simulink model "controller_estimator_test_static"  (R2016b)
settings: Solver=VariableStepAuto  StartTime=0.0  StopTime=200  RelTol=1e-3
values from neighbouring files (symbols this model uses):
  quat_cmd = quat_cmd/norm(quat_cmd)    [controller_estimator_test_init.m]
undefined symbols (not defined in the file or in its folder): Estimation_EKF, extended_kalman_filter_lib, fsw_params
libraries: dynamics_lib x2, pd_control_lib x1, aerolibutil x1, sensors_lib x1, sensor_processing x1
settings Model: Creator=sexymathemagician  LastModifiedBy=sexymathemagician

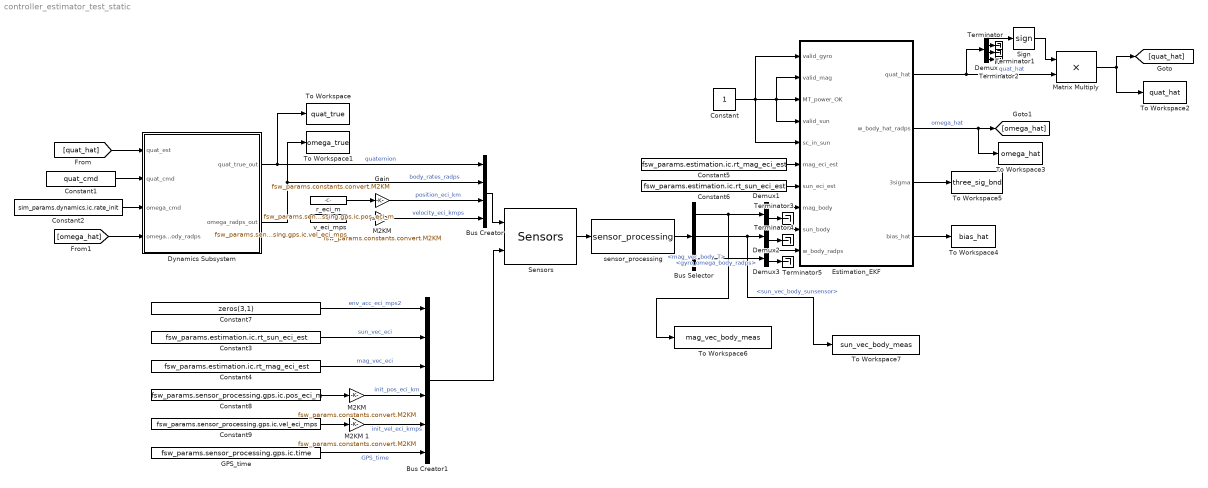
== system controller_estimator_test_static ==
  Bus Creator : BusCreator  Inputs=4
  Bus Creator1 : BusCreator  Inputs=6
  Bus Selector : BusSelector  OutputSignals=mag_vec_body_T,sun_vec_body_sunsensor,gyro_omega_body_radps
  Constant : Constant
  Constant1 : Constant  Value=quat_cmd
  Constant2 : Constant  Value=sim_params.dynamics.ic.rate_init
  Constant3 : Constant  Value=fsw_params.estimation.ic.rt_sun_eci_est
  Constant4 : Constant  Value=fsw_params.estimation.ic.rt_mag_eci_est
  Constant5 : Constant  Value=fsw_params.estimation.ic.rt_mag_eci_est
  Constant6 : Constant  Value=fsw_params.estimation.ic.rt_sun_eci_est
  Constant7 : Constant  Value=zeros(3,1)
  Constant8 : Constant  Value=fsw_params.sensor_processing.gps.ic.pos_eci_m
  Constant9 : Constant  Value=fsw_params.sensor_processing.gps.ic.vel_eci_mps
  Demux : Demux
  Demux1 : Demux  Outputs=[3 1]
  Demux2 : Demux  Outputs=[3 1]
  Demux3 : Demux  Outputs=[3 1]
  Dynamics Subsystem : Subsystem
  "Estimation_EKF " : Subsystem  AncestorBlock=extended_kalman_filter_lib/Estimation_EKF
  GPS_time : Constant  Value=fsw_params.sensor_processing.gps.ic.time
  Gain : Gain  Gain=fsw_params.constants.convert.M2KM
  M2KM : Gain  Gain=fsw_params.constants.convert.M2KM
  "M2KM " : Gain  Gain=fsw_params.constants.convert.M2KM
  M2KM 1 : Gain  Gain=fsw_params.constants.convert.M2KM
  Matrix Multiply : Product
  Sensors : sensors_lib/Sensors
      link override Bus Selector2: OutputSignals=sun_vec_eci,mag_vec_eci
  Sign : Signum
  Terminator{,1..5} (6 alike) : Terminator
  To Workspace : ToWorkspace  VariableName=quat_true  SaveFormat=Timeseries  SampleTime=-1
  To Workspace1 : ToWorkspace  VariableName=omega_true  SaveFormat=Timeseries  SampleTime=-1
  To Workspace2 : ToWorkspace  VariableName=quat_hat  SaveFormat=Timeseries  SampleTime=-1
  To Workspace3 : ToWorkspace  VariableName=omega_hat  SaveFormat=Timeseries  SampleTime=-1
  To Workspace4 : ToWorkspace  VariableName=bias_hat  SaveFormat=Timeseries  SampleTime=-1
  To Workspace5 : ToWorkspace  VariableName=three_sig_bnd  SaveFormat=Timeseries  SampleTime=-1
  To Workspace6 : ToWorkspace  VariableName=mag_vec_body_meas  SaveFormat=Timeseries  SampleTime=-1
  To Workspace7 : ToWorkspace  VariableName=sun_vec_body_meas  SaveFormat=Timeseries  SampleTime=-1
  r_eci_m : Constant  Value=fsw_params.sensor_processing.gps.ic.pos_eci_m
  sensor_processing : sensor_processing/sensor_processing
  v_eci_mps : Constant  Value=fsw_params.sensor_processing.gps.ic.vel_eci_mps
  wires:
  Constant/1 -> "Estimation_EKF "/5(sc_in_sun), "Estimation_EKF "/1(valid_gyro), "Estimation_EKF "/4("valid_sun "), "Estimation_EKF "/2(valid_mag), "Estimation_EKF "/3(MT_power_OK)
  "Estimation_EKF "/3(3sigma) -> To Workspace5/1
  "Estimation_EKF "/4(bias_hat) -> To Workspace4/1
  Dynamics Subsystem/1(quat_true_out) -> Bus Creator/1, To Workspace/1  "quaternion"
  Dynamics Subsystem/2(omega_radps_out) -> Bus Creator/2, To Workspace1/1  "body_rates_radps"
  [quat_hat] -> Dynamics Subsystem/1(quat_est)
  "Estimation_EKF "/2(w_body_hat_radps) -> To Workspace3/1, [omega_hat]  "omega_hat"
  [omega_hat] -> Dynamics Subsystem/4(omega_body_radps)
  Constant1/1 -> Dynamics Subsystem/2(quat_cmd)
  Constant2/1 -> Dynamics Subsystem/3("omega_cmd ")
  "Estimation_EKF "/1(quat_hat) -> Demux/1, Matrix Multiply/2  "quat_hat"
  Demux/2 -> Terminator/1
  Demux/3 -> Terminator1/1
  Demux/4 -> Terminator2/1
  Demux/1 -> Sign/1
  Sign/1 -> Matrix Multiply/1
  Sensors/1 -> sensor_processing/1
  sensor_processing/1 -> Bus Selector/1
  Bus Creator/1 -> Sensors/1
  Bus Selector/1 -> To Workspace6/1, Demux1/1  "<mag_vec_body_T>"
  Bus Selector/2 -> To Workspace7/1, Demux2/1  "<sun_vec_body_sunsensor>"
  Bus Selector/3 -> Demux3/1  "<gyro_omega_body_radps>"
  r_eci_m/1 -> Gain/1
  Constant4/1 -> Bus Creator1/3  "mag_vec_eci"
  Constant3/1 -> Bus Creator1/2  "sun_vec_eci"
  GPS_time/1 -> Bus Creator1/6  "GPS_time"
  Bus Creator1/1 -> Sensors/2
  Constant6/1 -> "Estimation_EKF "/7(sun_eci_est)
  Constant5/1 -> "Estimation_EKF "/6(mag_eci_est)
  Constant7/1 -> Bus Creator1/1  "env_acc_eci_mps2"
  Constant8/1 -> "M2KM "/1
  Constant9/1 -> M2KM 1/1
  Gain/1 -> Bus Creator/3  "position_eci_km"
  v_eci_mps/1 -> M2KM/1
  M2KM/1 -> Bus Creator/4  "velocity_eci_kmps"
  "M2KM "/1 -> Bus Creator1/4  "init_pos_eci_km"
  M2KM 1/1 -> Bus Creator1/5  "init_vel_eci_kmps"
  Demux1/1 -> "Estimation_EKF "/8(mag_body)
  Demux2/1 -> "Estimation_EKF "/9(sun_body)
  Demux3/1 -> "Estimation_EKF "/10(w_body_radps)
  Demux1/2 -> Terminator3/1
  Demux2/2 -> Terminator4/1
  Demux3/2 -> Terminator5/1
  Matrix Multiply/1 -> To Workspace2/1, [quat_hat]

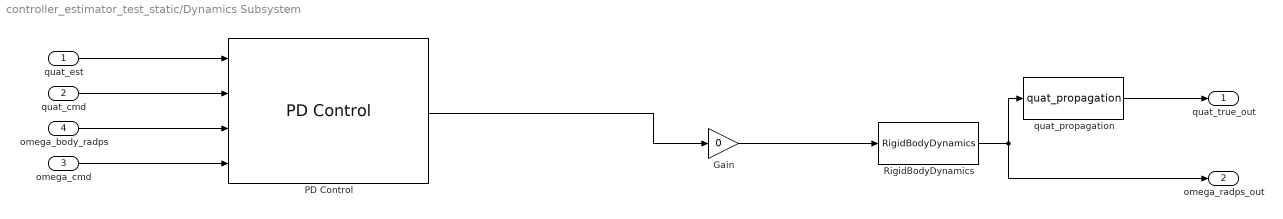
== system controller_estimator_test_static/Dynamics Subsystem ==
  quat_est : Inport
  quat_cmd : Inport  Port=2
  "omega_cmd " : Inport  Port=3
  omega_body_radps : Inport  Port=4
  Gain : Gain  Gain=0
  PD Control : pd_control_lib/PD Control
  RigidBodyDynamics : dynamics_lib/Dynamics/RigidBodyDynamics
  quat_propagation : dynamics_lib/Dynamics/quat_propagation
  quat_true_out : Outport
  omega_radps_out : Outport  Port=2
  wires:
  "omega_cmd "/1 -> PD Control/4
  quat_est/1 -> PD Control/1
  quat_cmd/1 -> PD Control/2
  omega_body_radps/1 -> PD Control/3
  RigidBodyDynamics/1 -> omega_radps_out/1, quat_propagation/1
  quat_propagation/1 -> quat_true_out/1
  PD Control/1 -> Gain/1
  Gain/1 -> RigidBodyDynamics/1

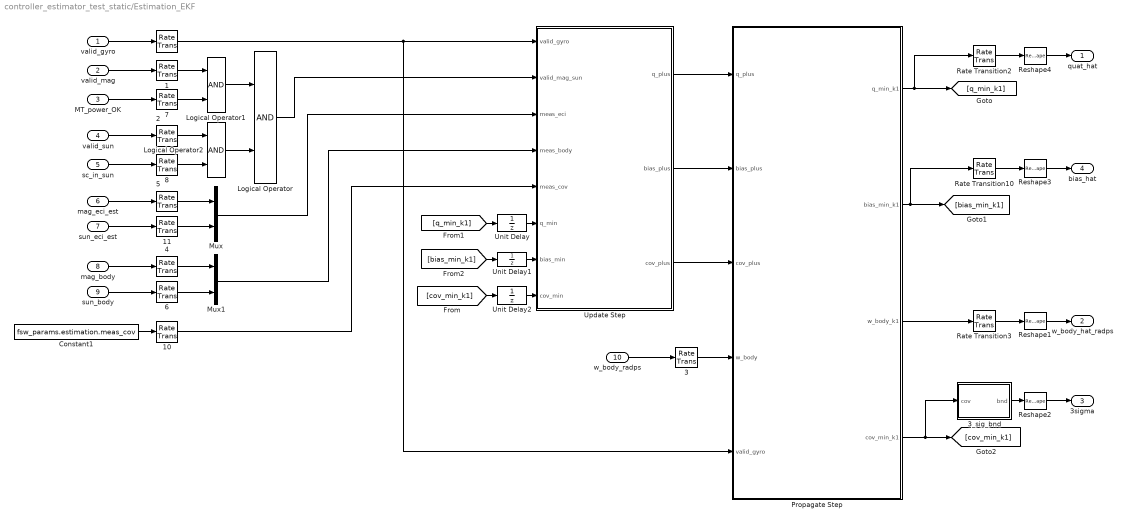
== system controller_estimator_test_static/Estimation_EKF  ==
  valid_gyro : Inport
  valid_mag : Inport  Port=2
  MT_power_OK : Inport  Port=3
  "valid_sun " : Inport  Port=4
  sc_in_sun : Inport  Port=5
  mag_eci_est : Inport  Port=6
  sun_eci_est : Inport  Port=7
  mag_body : Inport  Port=8
  sun_body : Inport  Port=9
  w_body_radps : Inport  Port=10
  " " : RateTransition  X0=fsw_params.estimation.ic.rt_valid_gyro  OutPortSampleTime=fsw_params.estimation.sample_time_s
  " 1" : RateTransition  X0=fsw_params.estimation.ic.rt_valid_mag  OutPortSampleTime=fsw_params.estimation.sample_time_s
  " 10" : RateTransition  X0=fsw_params.estimation.ic.rt_meas_cov  OutPortSampleTime=fsw_params.estimation.sample_time_s
  " 11" : RateTransition  X0=fsw_params.estimation.ic.rt_sun_eci_est  OutPortSampleTime=fsw_params.estimation.sample_time_s
  " 2" : RateTransition  X0=fsw_params.estimation.ic.rt_valid_sun  OutPortSampleTime=fsw_params.estimation.sample_time_s
  " 3" : RateTransition  X0=fsw_params.estimation.ic.rt_w_body_radps  OutPortSampleTime=fsw_params.estimation.sample_time_s
  " 4" : RateTransition  X0=fsw_params.estimation.ic.rt_mag_body  OutPortSampleTime=fsw_params.estimation.sample_time_s
  " 5" : RateTransition  X0=fsw_params.estimation.ic.rt_mag_eci_est  OutPortSampleTime=fsw_params.estimation.sample_time_s
  " 6" : RateTransition  X0=fsw_params.estimation.ic.rt_sun_body  OutPortSampleTime=fsw_params.estimation.sample_time_s
  " 7" : RateTransition  X0=fsw_params.estimation.ic.rt_mt_power_ok  OutPortSampleTime=fsw_params.estimation.sample_time_s
  " 8" : RateTransition  X0=fsw_params.estimation.ic.rt_sc_in_sun  OutPortSampleTime=fsw_params.estimation.sample_time_s
  "3_sig_bnd " : MATLAB Function  TreatAsAtomicUnit=on
  Constant1 : Constant  Value=fsw_params.estimation.meas_cov
  Logical Operator : Logic  AllPortsSameDT=off  OutDataTypeStr=boolean
  Logical Operator1 : Logic  AllPortsSameDT=off  OutDataTypeStr=boolean
  Logical Operator2 : Logic  AllPortsSameDT=off  OutDataTypeStr=boolean
  Mux : Mux  Inputs=2
  Mux1 : Mux  Inputs=2
  "Propagate Step " : Subsystem
  Rate Transition10 : RateTransition  X0=fsw_params.estimation.ic.bias_est_init
  Rate Transition2 : RateTransition  X0=fsw_params.estimation.ic.quat_est_init
  Rate Transition3 : RateTransition  X0=fsw_params.estimation.ic.rate_est_init
  Reshape{1..4} (4 alike) : Reshape  OutputDimensions=[3,1]
  Unit Delay : UnitDelay  InitialCondition=fsw_params.estimation.ic.quat_est_init  SampleTime=fsw_params.estimation.sample_time_s
  Unit Delay1 : UnitDelay  InitialCondition=fsw_params.estimation.ic.bias_est_init  SampleTime=fsw_params.estimation.sample_time_s
  Unit Delay2 : UnitDelay  InitialCondition=fsw_params.estimation.ic.error_cov  SampleTime=fsw_params.estimation.sample_time_s
  "Update Step " : Subsystem
  quat_hat : Outport
  w_body_hat_radps : Outport  Port=2
  3sigma : Outport  Port=3
  bias_hat : Outport  Port=4
  wires:
  Logical Operator2/1 -> Logical Operator/2
  Logical Operator1/1 -> Logical Operator/1
  " 2"/1 -> Logical Operator2/1
  " 8"/1 -> Logical Operator2/2
  sc_in_sun/1 -> " 8"/1
  " 1"/1 -> Logical Operator1/1
  " 7"/1 -> Logical Operator1/2
  MT_power_OK/1 -> " 7"/1
  Constant1/1 -> " 10"/1
  Unit Delay/1 -> "Update Step "/6(q_min)
  [q_min_k1] -> Unit Delay/1
  Unit Delay1/1 -> "Update Step "/7(bias_min)
  [bias_min_k1] -> Unit Delay1/1
  Unit Delay2/1 -> "Update Step "/8(cov_min)
  [cov_min_k1] -> Unit Delay2/1
  "3_sig_bnd "/1(bnd) -> Reshape2/1
  "Propagate Step "/4(cov_min_k1) -> "3_sig_bnd "/1(cov), [cov_min_k1]
  Rate Transition10/1 -> Reshape3/1
  Rate Transition3/1 -> Reshape1/1
  Rate Transition2/1 -> Reshape4/1
  Reshape4/1 -> quat_hat/1
  Reshape1/1 -> w_body_hat_radps/1
  Reshape2/1 -> 3sigma/1
  Reshape3/1 -> bias_hat/1
  " "/1 -> "Update Step "/1(valid_gyro), "Propagate Step "/5(valid_gyro)
  "Propagate Step "/3(w_body_k1) -> Rate Transition3/1
  "Propagate Step "/2(bias_min_k1) -> Rate Transition10/1, [bias_min_k1]
  "Propagate Step "/1(q_min_k1) -> Rate Transition2/1, [q_min_k1]
  " 10"/1 -> "Update Step "/5(meas_cov)
  Mux1/1 -> "Update Step "/4(meas_body)
  " 6"/1 -> Mux1/2
  " 4"/1 -> Mux1/1
  Mux/1 -> "Update Step "/3(meas_eci)
  " 11"/1 -> Mux/2
  " 5"/1 -> Mux/1
  " 3"/1 -> "Propagate Step "/4(w_body)
  Logical Operator/1 -> "Update Step "/2(valid_mag_sun)
  sun_eci_est/1 -> " 11"/1
  sun_body/1 -> " 6"/1
  mag_eci_est/1 -> " 5"/1
  mag_body/1 -> " 4"/1
  w_body_radps/1 -> " 3"/1
  "valid_sun "/1 -> " 2"/1
  valid_mag/1 -> " 1"/1
  valid_gyro/1 -> " "/1
  "Update Step "/3(cov_plus) -> "Propagate Step "/3(cov_plus)
  "Update Step "/2(bias_plus) -> "Propagate Step "/2(bias_plus)
  "Update Step "/1(q_plus) -> "Propagate Step "/1(q_plus)

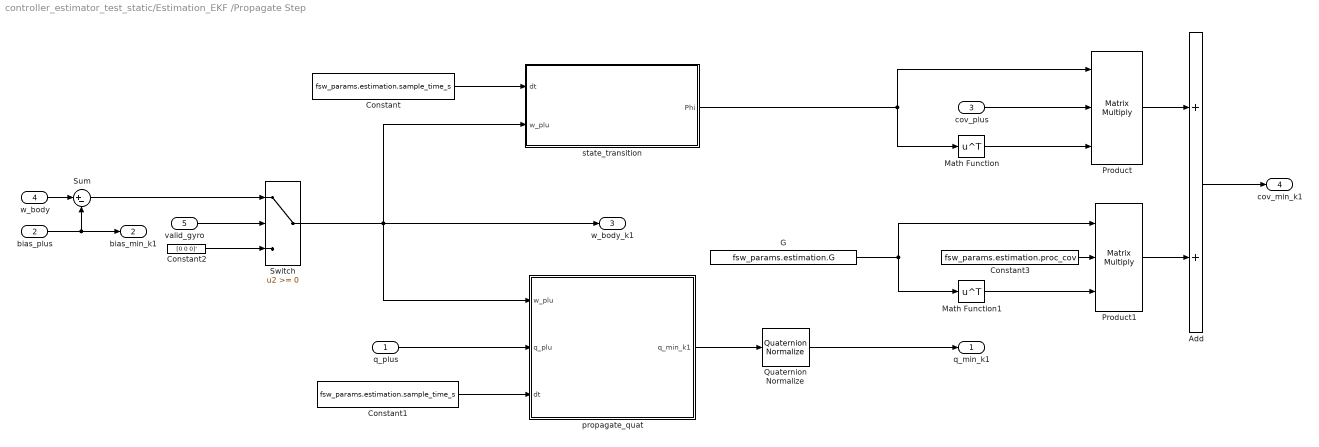
== system controller_estimator_test_static/Estimation_EKF /Propagate Step  ==
  q_plus : Inport
  bias_plus : Inport  Port=2
  cov_plus : Inport  Port=3
  w_body : Inport  Port=4
  valid_gyro : Inport  Port=5
  Add : Sum
  Constant : Constant  Value=fsw_params.estimation.sample_time_s
  Constant1 : Constant  Value=fsw_params.estimation.sample_time_s
  Constant2 : Constant  Value=[0 0 0]'
  Constant3 : Constant  Value=fsw_params.estimation.proc_cov
  G : Constant  Value=fsw_params.estimation.G
  Math Function : Math  Operator=transpose  SaturateOnIntegerOverflow=on
  Math Function1 : Math  Operator=transpose  SaturateOnIntegerOverflow=on
  Product : Product  Inputs=***  Multiplication=Matrix(*)  RndMeth=Zero
  Product1 : Product  Inputs=***  Multiplication=Matrix(*)  RndMeth=Zero
  Quaternion Normalize : aerolibutil/Quaternion Normalize
  Sum : Sum  Inputs=|+-
  Switch : Switch
  propagate_quat : MATLAB Function  TreatAsAtomicUnit=on
  state_transition : MATLAB Function  TreatAsAtomicUnit=on
  q_min_k1 : Outport
  bias_min_k1 : Outport  Port=2
  w_body_k1 : Outport  Port=3
  cov_min_k1 : Outport  Port=4
  wires:
  Sum/1 -> Switch/1
  Constant2/1 -> Switch/3
  state_transition/1(Phi) -> Product/1, Math Function/1
  Add/1 -> cov_min_k1/1
  Math Function/1 -> Product/3
  cov_plus/1 -> Product/2
  G/1 -> Math Function1/1, Product1/1
  Math Function1/1 -> Product1/3
  Constant3/1 -> Product1/2
  Product/1 -> Add/1
  Product1/1 -> Add/2
  Quaternion Normalize/1 -> q_min_k1/1
  propagate_quat/1(q_min_k1) -> Quaternion Normalize/1
  Switch/1 -> state_transition/2(w_plu), propagate_quat/1(w_plu), w_body_k1/1
  bias_plus/1 -> Sum/2, bias_min_k1/1
  w_body/1 -> Sum/1
  valid_gyro/1 -> Switch/2
  Constant1/1 -> propagate_quat/3(dt)
  Constant/1 -> state_transition/1(dt)
  q_plus/1 -> propagate_quat/2(q_plu)

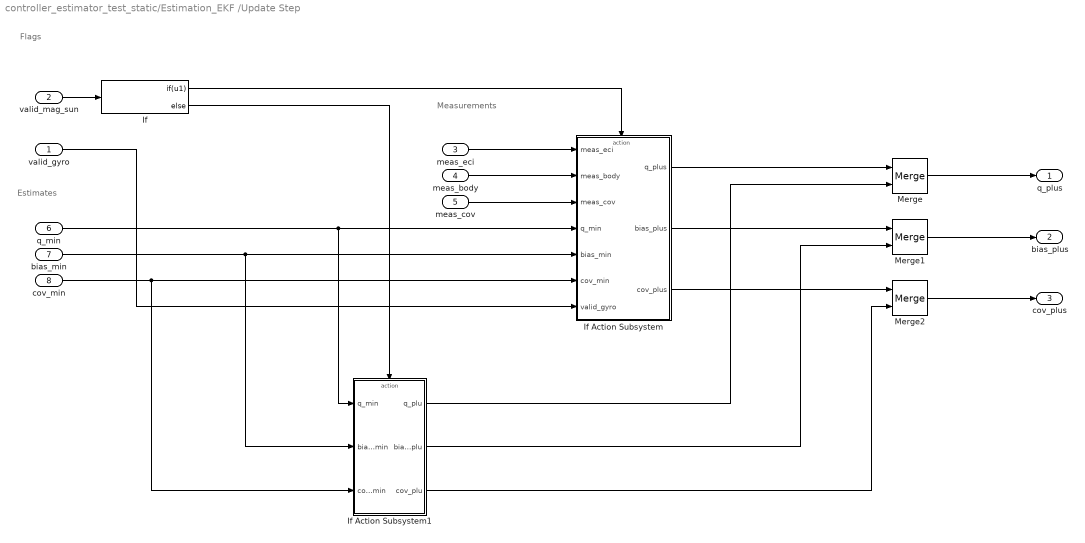
== system controller_estimator_test_static/Estimation_EKF /Update Step  ==
  note: Measurements
  note: Estimates
  note: Flags
  valid_gyro : Inport
  valid_mag_sun : Inport  Port=2
  meas_eci : Inport  Port=3
  meas_body : Inport  Port=4
  meas_cov : Inport  Port=5
  q_min : Inport  Port=6
  bias_min : Inport  Port=7
  cov_min : Inport  Port=8
  If : If  IfExpression=u1
  If Action Subsystem : Subsystem  TreatAsAtomicUnit=on
  If Action Subsystem1 : Subsystem  TreatAsAtomicUnit=on
  Merge : Merge
  Merge1 : Merge
  Merge2 : Merge
  q_plus : Outport
  bias_plus : Outport  Port=2
  cov_plus : Outport  Port=3
  wires:
  If/2 -> If Action Subsystem1/Action
  If/1 -> If Action Subsystem/Action
  If Action Subsystem/3(cov_plus) -> Merge2/1
  If Action Subsystem/2(bias_plus) -> Merge1/1
  If Action Subsystem/1(q_plus) -> Merge/1
  valid_gyro/1 -> If Action Subsystem/7(valid_gyro)
  meas_cov/1 -> If Action Subsystem/3(meas_cov)
  meas_body/1 -> If Action Subsystem/2("meas_body ")
  meas_eci/1 -> If Action Subsystem/1(meas_eci)
  If Action Subsystem1/3(cov_plu) -> Merge2/2
  If Action Subsystem1/2(bias_plu) -> Merge1/2
  If Action Subsystem1/1(q_plu) -> Merge/2
  Merge2/1 -> cov_plus/1
  Merge1/1 -> bias_plus/1
  Merge/1 -> q_plus/1
  cov_min/1 -> If Action Subsystem/6(cov_min), If Action Subsystem1/3(cov_min)
  bias_min/1 -> If Action Subsystem/5(bias_min), If Action Subsystem1/2(bias_min)
  q_min/1 -> If Action Subsystem/4("q_min "), If Action Subsystem1/1(q_min)
  valid_mag_sun/1 -> If/1

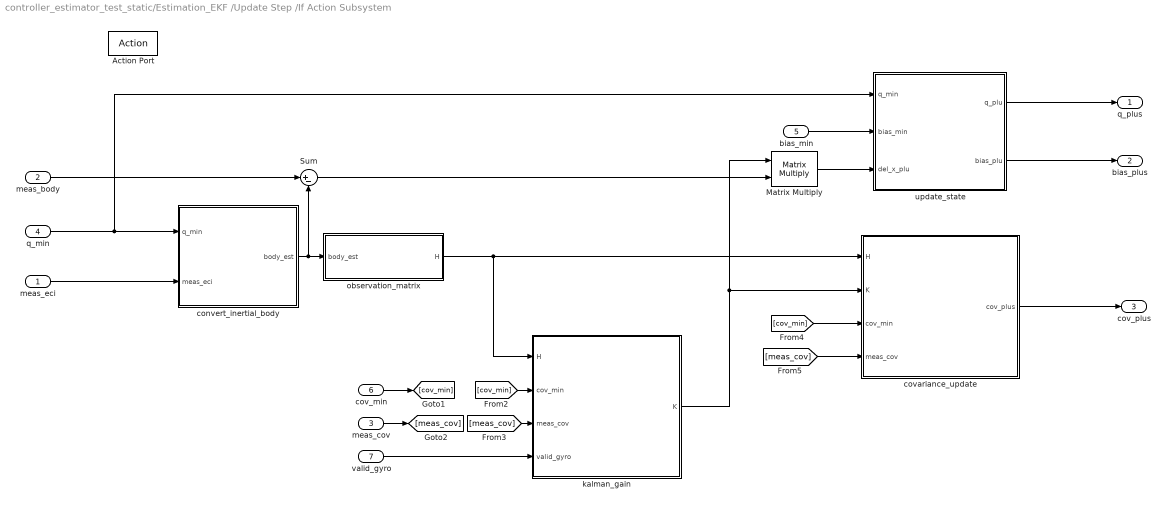
== system controller_estimator_test_static/Estimation_EKF /Update Step /If Action Subsystem ==
  meas_eci : Inport
  "meas_body " : Inport  Port=2
  meas_cov : Inport  Port=3
  "q_min " : Inport  Port=4
  bias_min : Inport  Port=5
  cov_min : Inport  Port=6
  valid_gyro : Inport  Port=7
  Action Port : ActionPort  ActionType=then
  Matrix Multiply : Product  Multiplication=Matrix(*)
  Sum : Sum  Inputs=|+-
  convert_inertial_body : MATLAB Function  TreatAsAtomicUnit=on
  covariance_update : MATLAB Function  TreatAsAtomicUnit=on
  kalman_gain : MATLAB Function  TreatAsAtomicUnit=on
  observation_matrix : MATLAB Function  TreatAsAtomicUnit=on
  "update_state " : MATLAB Function  TreatAsAtomicUnit=on
  q_plus : Outport
  bias_plus : Outport  Port=2
  cov_plus : Outport  Port=3
  wires:
  "q_min "/1 -> convert_inertial_body/1(q_min), "update_state "/1(q_min)
  [meas_cov] -> covariance_update/4(meas_cov)
  [cov_min] -> covariance_update/3(cov_min)
  [meas_cov] -> kalman_gain/3(meas_cov)
  meas_cov/1 -> [meas_cov]
  [cov_min] -> kalman_gain/2(cov_min)
  cov_min/1 -> [cov_min]
  Matrix Multiply/1 -> "update_state "/3(del_x_plu)
  Sum/1 -> Matrix Multiply/2
  "update_state "/2(bias_plu) -> bias_plus/1
  "update_state "/1(q_plu) -> q_plus/1
  bias_min/1 -> "update_state "/2(bias_min)
  covariance_update/1(cov_plus) -> cov_plus/1
  kalman_gain/1(K) -> covariance_update/2(K), Matrix Multiply/1
  "meas_body "/1 -> Sum/1
  observation_matrix/1(H) -> kalman_gain/1(H), covariance_update/1(H)
  valid_gyro/1 -> kalman_gain/4(valid_gyro)
  meas_eci/1 -> convert_inertial_body/2(meas_eci)
  convert_inertial_body/1(body_est) -> observation_matrix/1(body_est), Sum/2

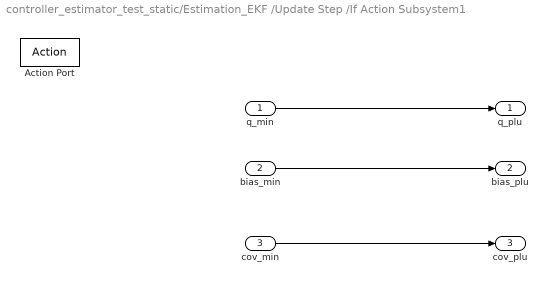
== system controller_estimator_test_static/Estimation_EKF /Update Step /If Action Subsystem1 ==
  q_min : Inport
  bias_min : Inport  Port=2
  cov_min : Inport  Port=3
  Action Port : ActionPort  ActionType=else
  q_plu : Outport
  bias_plu : Outport  Port=2
  cov_plu : Outport  Port=3
  wires:
  cov_min/1 -> cov_plu/1
  bias_min/1 -> bias_plu/1
  q_min/1 -> q_plu/1

== matlab function controller_estimator_test_static/Estimation_EKF /Update Step /If Action Subsystem/convert_inertial_body ==
  data: q_min input; body_est output; meas_eci input
function body_est = convert_inertial_body(q_min,meas_eci)

rotation_matrix = att(q_min);
body_est = blkdiag(rotation_matrix,rotation_matrix)*meas_eci;

end

function dcm = att(q)
dcm = [q(1)^2 + q(2)^2 - q(3)^2 - q(4)^2,   2*(q(2)*q(3)+q(1)*q(4)),    2*(q(2)*q(4) - q(1)*q(3));
        2*(q(2)*q(3) - q(1)*q(4)),          q(1)^2-q(2)^2+q(3)^2-q(4)^2,    2*(q(3)*q(4) + q(1)*q(2));
        2*(q(2)*q(4)+q(1)*q(3)),            2*(q(3)*q(4)-q(1)*q(2)),        q(1)^2-q(2)^2-q(3)^2+q(4)^2];
end

== matlab function controller_estimator_test_static/Estimation_EKF /Update Step /If Action Subsystem/covariance_update ==
  data: H input; cov_plus output; K input; cov_min input; meas_cov input
function cov_plus = covariance_update(H,K,cov_min,meas_cov)


 KHI = (K*H - eye(6));
 cov_plus = KHI*cov_min*KHI' + K*meas_cov*K';


end

== matlab function controller_estimator_test_static/Estimation_EKF /Update Step /If Action Subsystem/kalman_gain ==
  data: H input; K output; cov_min input; meas_cov input; valid_gyro input
function K = kalman_gain(H,cov_min,meas_cov,valid_gyro)

K = cov_min*H'/(H*cov_min*H' + meas_cov);

% zero off part of gain if gyro reading is invalid

if valid_gyro == 0
    K(4:6,:) = zeros(3,6);
end


end

== matlab function controller_estimator_test_static/Estimation_EKF /Update Step /If Action Subsystem/observation_matrix ==
  data: body_est input; H output
function H = observation_matrix(body_est)

H = [  skew(body_est(1:3))     zeros(3);
       skew(body_est(4:6))     zeros(3)];

end

function S = skew(v)
S = [0  -v(3)   v(2);
    v(3)    0   -v(1);
    -v(2)   v(1)    0];
end

== matlab function controller_estimator_test_static/Estimation_EKF /Update Step /If Action Subsystem/update_state  ==
  data: q_min input size=4; q_plu output size=4; bias_min input size=3; del_x_plu input size=6; bias_plu output size=3
function [q_plu,bias_plu] = update_state(q_min,bias_min,del_x_plu)
%#codegen

% select out bias
bias_plu = bias_min + del_x_plu(4:6);

q_plu = quat_update(del_x_plu(1:3),q_min);

end


function q_hat_pk = quat_update(del_apk, q_hat_mk)
%#codegen
%q_hat_pk = quat_multiply([sqrt(1-norm(del_apk/2)); del_apk/2], q_hat_mk);
q_hat_pk = quat_multiply([1; del_apk/2], q_hat_mk);

end

function q2 = quat_multiply(dq,q1)
%#codegen

q2 = quatmultiply(q1',dq')';
end

== matlab function controller_estimator_test_static/Estimation_EKF /Propagate Step /state_transition ==
  data: dt input; w_plu input; Phi output
function Phi = state_transition(dt,w_plu)

Phi = state_transition_matrix(w_plu,dt);

end

function phi = state_transition_matrix(w, dt)
%#codegen

w_n = norm(w);
w_skew = skew(w);

if w_n < 1e-14
    phi = [ eye(3) -eye(3)*dt;
            zeros(3,3) eye(3)];
else
    Phi_11 = eye(3) - w_skew*sin(w_n*dt)/w_n + w_skew^2*(1 - cos(w_n*dt))/w_n^2;
    
    Phi_12 = w_skew*(1 - cos(w_n*dt))/w_n^2 - eye(3)*dt - w_skew^2*(w_n*dt - sin(w_n*dt))/w_n^3;
    
    Phi_21 = zeros(3,3);
    
    Phi_22 = eye(3);
    
    phi = [ Phi_11 Phi_12;
            Phi_21 Phi_22];
end
end

function S = skew(v)
S = [0  -v(3)   v(2);
    v(3)    0   -v(1);
    -v(2)   v(1)    0];
end

== matlab function controller_estimator_test_static/Estimation_EKF /Propagate Step /propagate_quat ==
  data: w_plu input; q_min_k1 output; q_plu input; dt input
function q_min_k1 = propagate_quat(w_plu,q_plu,dt)

q_min_k1 = omega_matrix(w_plu,dt)*q_plu;

end

function omega = omega_matrix(w, dt)
w_n = norm(w);

if w_n < 1e-14
    Psi = 0*w;
else
    Psi = sin(1/2*w_n*dt)/w_n*w;
end

Psi_skew = skew(Psi);

omega = [cos(1/2*w_n*dt)*eye(3) - Psi_skew      Psi;
        -Psi'                                   cos(1/2*w_n*dt)];

T = [zeros(3,1) eye(3);
    1       zeros(1,3)];

omega = T'*omega*T;
end

function S = skew(v)
S = [0  -v(3)   v(2);
    v(3)    0   -v(1);
    -v(2)   v(1)    0];
end

== matlab function controller_estimator_test_static/Estimation_EKF /3_sig_bnd  ==
  data: cov input; bnd output
function bnd =  three_sig_bnd(cov)

bnd = cov;
